simulink model "ej"  (R2019a)
settings: Solver=VariableStepAuto  StartTime=0.0  StopTime=5  RelTol=1e-3
settings Model: Creator=cmparedes  LastModifiedBy=cmparedes

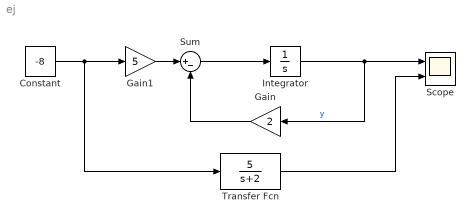
== system ej ==
  Constant : Constant  Value=-8
  Gain : Gain  Gain=2
  Gain1 : Gain  Gain=5
  Integrator : Integrator
  Scope : Scope  NumInputPorts=2
  Sum : Sum  Inputs=|+-
  Transfer Fcn : TransferFcn  Numerator=[5]  Denominator=[1 2]
  wires:
  Sum/1 -> Integrator/1
  Gain1/1 -> Sum/1
  Gain/1 -> Sum/2
  Integrator/1 -> Scope/1, Gain/1  "y"
  Constant/1 -> Transfer Fcn/1, Gain1/1
  Transfer Fcn/1 -> Scope/2
